simulink model "FilteredX_LMS_ANC"  (R2020a)
settings: Solver=FixedStepDiscrete  StartTime=0.0  StopTime=10  RelTol=1e-3
libraries: dspsrcs4 x1, dspadpt3 x1
settings Model: Creator=The MathWorks, Inc.  LastModifiedBy=Dell
settings DataIOCC: ReturnWorkspaceOutputs=off
settings DebuggingCC: ArithmeticOperatorsInVariantConditions=warning
settings SFSimCC: CustomCodeUndefinedFunction=UseInterfaceOnly

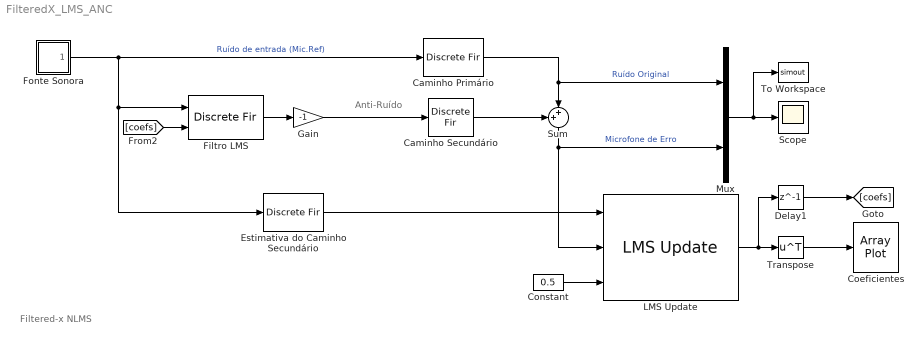
== system FilteredX_LMS_ANC ==
  note: Filtered-x NLMS
  note: Anti-Ruído
  Caminho Primário : DiscreteFir  Coefficients=conv([0.5 0.5 -.3 -.3 -.2 -.2],[.1 -.1 .2 -.2 .3 -.3 .15 -.15])
  Caminho Secundário : DiscreteFir  Coefficients=[0.5 0.5 -.3 -.3 -.2 -.2]
  Coeficientes : ArrayPlot
  Constant : Constant  Value=0.5
  Delay1 : Delay  DelayLength=1
  Estimativa do Caminho Secundário : DiscreteFir  Coefficients="[0.466  0.533  -0.257  -0.274  -0.231  -0.175]"
  Filtro LMS : DiscreteFir  CoefSource=Input port
      settings: InputPortMap=u0,u1
  Fonte Sonora : Subsystem
  Gain : Gain  Gain=-1
  LMS Update : dspadpt3/LMS Update  Method=Normalized LMS  Length=100  StepSizeSource=Input port  StepSize=0.1  LeakageFactor=1.0  InitialConditions=0  EnableAdaptInput=off  EnableResetInput=off  SimulateUsing=Interpreted execution
      settings: SourceProductBaseCode=DS
  Mux : Mux  Inputs=2
  Scope : Scope
  Sum : Sum  Inputs=++|
  To Workspace : ToWorkspace  VariableName=simout  SaveFormat=Timeseries  SampleTime=-1
  Transpose : Math  Operator=transpose  SignedPower=on  SaturateOnIntegerOverflow=on
  wires:
  Gain/1 -> Caminho Secundário/1
  Mux/1 -> To Workspace/1, Scope/1
  Estimativa do Caminho Secundário/1 -> LMS Update/1
  Delay1/1 -> [coefs]
  Caminho Secundário/1 -> Sum/1
  Transpose/1 -> Coeficientes/1
  [coefs] -> Filtro LMS/2
  Caminho Primário/1 -> Mux/1, Sum/2  "Ruído Original"
  Constant/1 -> LMS Update/3
  Filtro LMS/1 -> Gain/1
  Fonte Sonora/1(Out1) -> Estimativa do Caminho Secundário/1, Filtro LMS/1, Caminho Primário/1  "Ruído de entrada (Mic.Ref)"
  LMS Update/1 -> Transpose/1, Delay1/1
  Sum/1 -> Mux/2, LMS Update/2  "Microfone de Erro"

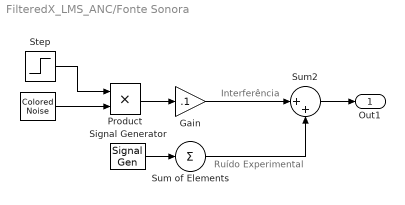
== system FilteredX_LMS_ANC/Fonte Sonora ==
  note: Interferência
  note: Ruído Experimental
  " " : dspsrcs4/Colored Noise  Color=white  InverseFrequencyPower=1  BoundedOutput=off  NumChannels=1  OutputDataType=double  SamplesPerFrame=1  SampleTime=1/8000  RandomStream=mt19937ar with seed  Seed=randi(1000)  SimulateUsing=Interpreted execution
      settings: SourceProductBaseCode=DS
  Gain : Gain  Gain=.1
  Product : Product
  Signal Generator : SignalGenerator  Amplitude=10 *[.15 1.8 1.2 2 1.3 .2 .3 .05 .01]  Frequency=[50 80 100 120 150 220 280 400 500]
  Step : Step  Time=0  SampleTime=0
  Sum of Elements : Sum  Inputs=+
  Sum2 : Sum  Inputs=|++
  Out1 : Outport  VectorParamsAs1DForOutWhenUnconnected=off
  wires:
  " "/1 -> Product/2
  Sum2/1 -> Out1/1
  Sum of Elements/1 -> Sum2/2
  Gain/1 -> Sum2/1
  Signal Generator/1 -> Sum of Elements/1
  Step/1 -> Product/1
  Product/1 -> Gain/1
